simulink model "test"  (R2023b)
settings: Solver=VariableStepAuto  StartTime=0.0  StopTime=0.5  RelTol=1e-3
libraries: spsFourierLib x2
settings Model: Creator=86134  LastModifiedBy=86134
settings OptimizationCC: ReuseModelBlockBuffer=off

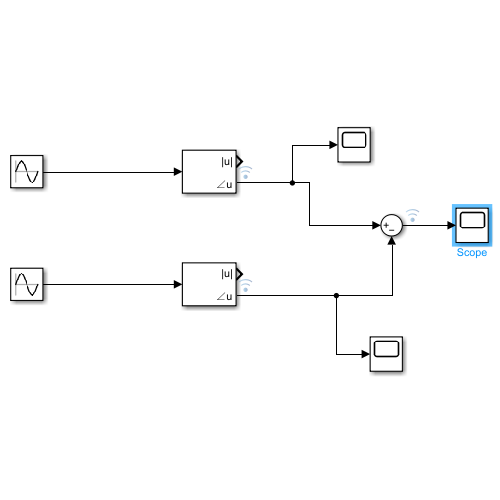
[thumbnail: Simulink's stored preview of the top-level diagram]
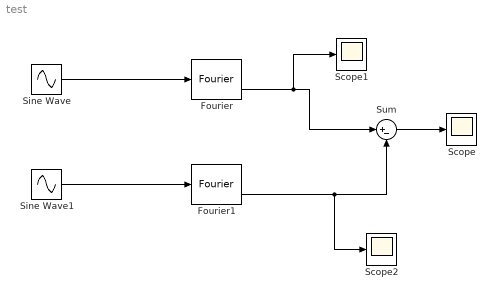
== system test ==
  Fourier : spsFourierLib/Fourier  Freq=4  n=1  InInit=[0, 0]  Ts=0
  Fourier1 : spsFourierLib/Fourier  Freq=4  n=1  InInit=[0, 0]  Ts=0
  Scope : Scope
  Scope1 : Scope
  Scope2 : Scope
  Sine Wave : Sin  Frequency=4*2*pi  Phase=pi/2  SampleTime=0
  Sine Wave1 : Sin  Frequency=4*2*pi  SampleTime=0
  Sum : Sum  Inputs=|+-
  wires:
  Sine Wave/1 -> Fourier/1
  Sine Wave1/1 -> Fourier1/1
  Fourier/2 -> Scope1/1, Sum/1
  Fourier1/2 -> Scope2/1, Sum/2
  Sum/1 -> Scope/1
